simulink model "motorised_pid_bob_system"  (R2025b)
settings: Solver=FixedStepAuto  StartTime=0.0  StopTime=20  FixedStep=1e-4  RelTol=1e-3
values from neighbouring files (symbols this model uses):
  c = Simulink.Parameter    [motorised_BoB_system_with_PID.m]
  g = Simulink.Parameter    [motorised_BoB_system_with_PID.m]
  J_beam = Simulink.Parameter    [motorised_BoB_system_with_PID.m]
  J_motor = Simulink.Parameter    [dc_drives_system_parameter_declaraction.m]    (also in motorised_BoB_system_with_PID.m)
  k_e = Simulink.Parameter    [dc_drives_system_parameter_declaraction.m]    (also in motorised_BoB_system_with_PID.m)
  k_t = Simulink.Parameter    [dc_drives_system_parameter_declaraction.m]    (also in motorised_BoB_system_with_PID.m)
  KDpid = Simulink.Parameter    [motorised_BoB_system_with_PID.m]
  kFrs = Simulink.Parameter    [dc_drives_system_parameter_declaraction.m]
  KIpid = Simulink.Parameter    [motorised_BoB_system_with_PID.m]
  KPpid = Simulink.Parameter    [motorised_BoB_system_with_PID.m]
  L_a = Simulink.Parameter    [dc_drives_system_parameter_declaraction.m]    (also in motorised_BoB_system_with_PID.m)
  l_beam = Simulink.Parameter    [motorised_BoB_system_with_PID.m]
  m_ball = Simulink.Parameter    [motorised_BoB_system_with_PID.m]
  R_a = Simulink.Parameter    [dc_drives_system_parameter_declaraction.m]    (also in motorised_BoB_system_with_PID.m)
  r_ball = Simulink.Parameter    [motorised_BoB_system_with_PID.m]
  W_ci = Simulink.Parameter    [dc_drives_system_parameter_declaraction.m]
  W_cq = Simulink.Parameter    [dc_drives_system_parameter_declaraction.m]
  W_cw = Simulink.Parameter    [dc_drives_system_parameter_declaraction.m]
undefined symbols (not defined in the file or in its folder): L, R
settings Model: Creator=fycce  LastModifiedBy=fycce

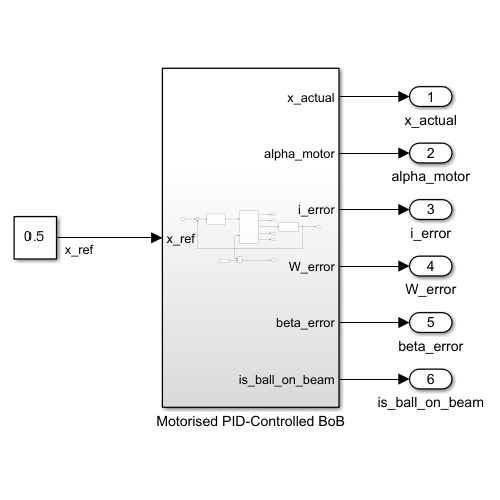
[thumbnail: Simulink's stored preview of the top-level diagram]
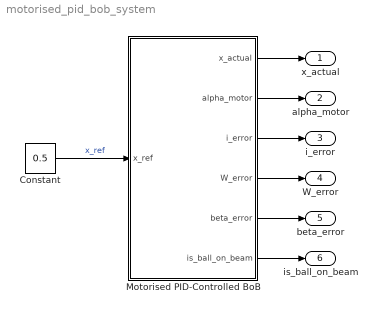
== system motorised_pid_bob_system ==
  Constant : Constant  Value=0.5
  Motorised PID-Controlled BoB : Subsystem
  x_actual : Outport
  alpha_motor : Outport  Port=2
  i_error : Outport  Port=3
  W_error : Outport  Port=4
  beta_error : Outport  Port=5
  is_ball_on_beam : Outport  Port=6
  wires:
  Constant/1 -> Motorised PID-Controlled BoB/1(x_ref)  "x_ref"
  Motorised PID-Controlled BoB/1(x_actual) -> x_actual/1
  Motorised PID-Controlled BoB/2(alpha_motor) -> alpha_motor/1
  Motorised PID-Controlled BoB/3(i_error) -> i_error/1
  Motorised PID-Controlled BoB/4(W_error) -> W_error/1
  Motorised PID-Controlled BoB/5(beta_error) -> beta_error/1
  Motorised PID-Controlled BoB/6(is_ball_on_beam) -> is_ball_on_beam/1

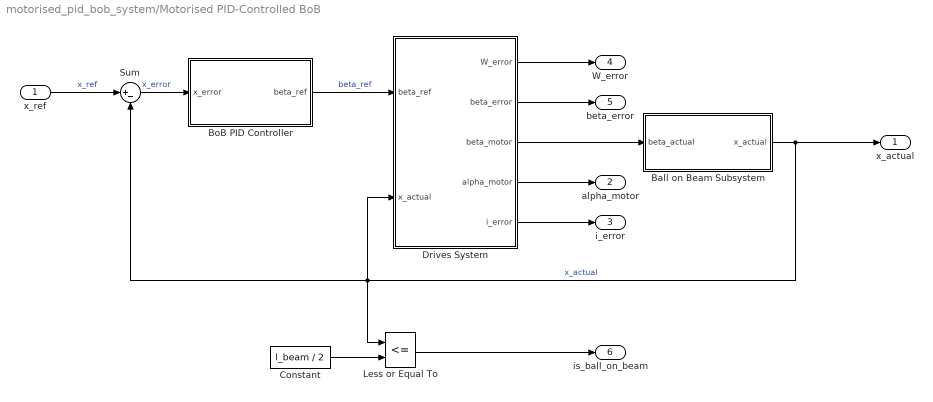
== system motorised_pid_bob_system/Motorised PID-Controlled BoB ==
  x_ref : Inport
  Ball on Beam Subsystem : Subsystem
  BoB PID Controller : Subsystem
  Constant : Constant  Value=l_beam / 2
  Drives System : Subsystem
  Less or Equal To : RelationalOperator  Operator=<=  OutDataTypeStr=boolean  RndMeth=Simplest  InputSameDT=off
  Sum : Sum  Inputs=|+-
  x_actual : Outport
  alpha_motor : Outport  Port=2
  i_error : Outport  Port=3
  W_error : Outport  Port=4
  beta_error : Outport  Port=5
  is_ball_on_beam : Outport  Port=6
  wires:
  Ball on Beam Subsystem/1(x_actual) -> x_actual/1, Less or Equal To/1, Sum/2, Drives System/2(x_actual)  "x_actual"
  Drives System/2(beta_error) -> beta_error/1
  Sum/1 -> BoB PID Controller/1(x_error)  "x_error"
  x_ref/1 -> Sum/1  "x_ref"
  Drives System/1(W_error) -> W_error/1
  Drives System/3(beta_motor) -> Ball on Beam Subsystem/1(beta_actual)
  Drives System/4(alpha_motor) -> alpha_motor/1
  BoB PID Controller/1(beta_ref) -> Drives System/1(beta_ref)  "beta_ref"
  Drives System/5(i_error) -> i_error/1
  Constant/1 -> Less or Equal To/2
  Less or Equal To/1 -> is_ball_on_beam/1

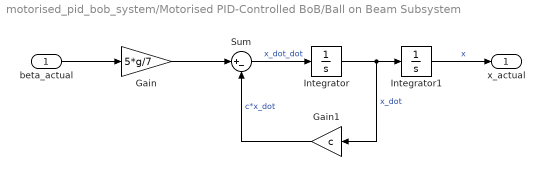
== system motorised_pid_bob_system/Motorised PID-Controlled BoB/Ball on Beam Subsystem ==
  beta_actual : Inport
  Gain : Gain  Gain=5*g/7
  Gain1 : Gain  Gain=c
  Integrator : Integrator
  Integrator1 : Integrator
  Sum : Sum  Inputs=|+-
  x_actual : Outport
  wires:
  Integrator1/1 -> x_actual/1  "x"
  beta_actual/1 -> Gain/1
  Integrator/1 -> Integrator1/1, Gain1/1  "x_dot"
  Gain/1 -> Sum/1
  Sum/1 -> Integrator/1  "x_dot_dot"
  Gain1/1 -> Sum/2  "c*x_dot"

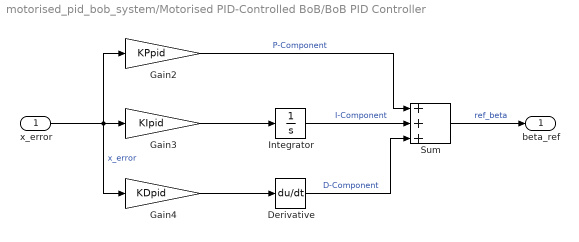
== system motorised_pid_bob_system/Motorised PID-Controlled BoB/BoB PID Controller ==
  x_error : Inport
  Derivative : Derivative
  Gain2 : Gain  Gain=KPpid
  Gain3 : Gain  Gain=KIpid
  Gain4 : Gain  Gain=KDpid
  Integrator : Integrator
  Sum : Sum  Inputs=+++
  beta_ref : Outport
  wires:
  Gain2/1 -> Sum/1  "P-Component"
  Integrator/1 -> Sum/2  "I-Component"
  Gain3/1 -> Integrator/1
  Sum/1 -> beta_ref/1  "ref_beta"
  Derivative/1 -> Sum/3  "D-Component"
  x_error/1 -> Gain4/1, Gain3/1, Gain2/1  "x_error"
  Gain4/1 -> Derivative/1

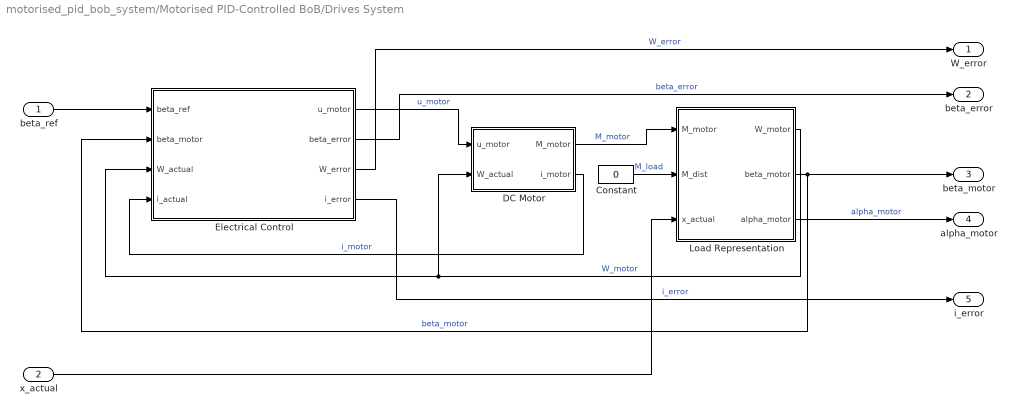
== system motorised_pid_bob_system/Motorised PID-Controlled BoB/Drives System ==
  beta_ref : Inport
  x_actual : Inport  Port=2
  Constant : Constant  Value=0
  DC Motor : Subsystem
  Electrical Control : Subsystem
  Load Representation : Subsystem
  W_error : Outport
  beta_error : Outport  Port=2
  beta_motor : Outport  Port=3
  alpha_motor : Outport  Port=4
  i_error : Outport  Port=5
  wires:
  DC Motor/2(i_motor) -> Electrical Control/4(i_actual)  "i_motor"
  Electrical Control/3(W_error) -> W_error/1  "W_error"
  Electrical Control/2(beta_error) -> beta_error/1  "beta_error"
  Load Representation/2(beta_motor) -> Electrical Control/2(beta_motor), beta_motor/1  "beta_motor"
  Electrical Control/1(u_motor) -> DC Motor/1(u_motor)  "u_motor"
  Load Representation/1(W_motor) -> Electrical Control/3(W_actual), DC Motor/2(W_actual)  "W_motor"
  DC Motor/1(M_motor) -> Load Representation/1(M_motor)  "M_motor"
  beta_ref/1 -> Electrical Control/1(beta_ref)
  Electrical Control/4(i_error) -> i_error/1  "i_error"
  Load Representation/3(alpha_motor) -> alpha_motor/1  "alpha_motor"
  Constant/1 -> Load Representation/2(M_dist)  "M_load"
  x_actual/1 -> Load Representation/3(x_actual)

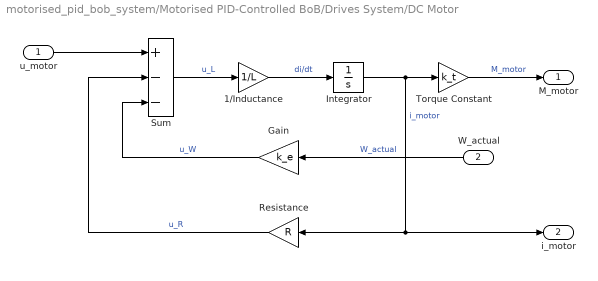
== system motorised_pid_bob_system/Motorised PID-Controlled BoB/Drives System/DC Motor ==
  u_motor : Inport
  W_actual : Inport  Port=2
  1/Inductance : Gain  Gain=1/L
  Gain : Gain  Gain=k_e
  Integrator : Integrator
  Resistance : Gain  Gain=R
  Sum : Sum  Inputs=+--
  Torque Constant : Gain  Gain=k_t
  M_motor : Outport
  i_motor : Outport  Port=2
  wires:
  u_motor/1 -> Sum/1
  Sum/1 -> 1/Inductance/1  "u_L"
  1/Inductance/1 -> Integrator/1  "di/dt"
  Integrator/1 -> i_motor/1, Resistance/1, Torque Constant/1  "i_motor"
  Torque Constant/1 -> M_motor/1  "M_motor"
  Resistance/1 -> Sum/2  "u_R"
  Gain/1 -> Sum/3  "u_W"
  W_actual/1 -> Gain/1  "W_actual"

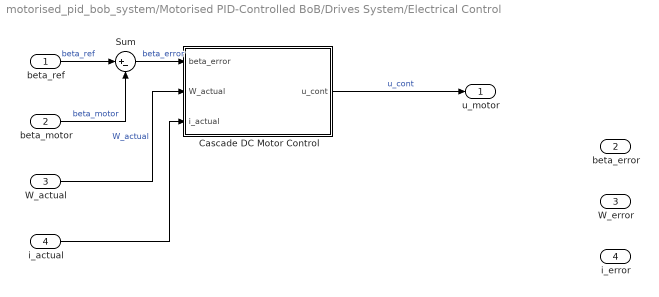
== system motorised_pid_bob_system/Motorised PID-Controlled BoB/Drives System/Electrical Control ==
  beta_ref : Inport
  beta_motor : Inport  Port=2
  W_actual : Inport  Port=3
  i_actual : Inport  Port=4
  Cascade DC Motor Control : Subsystem
  Sum : Sum  Inputs=|+-
  u_motor : Outport
  beta_error : Outport  Port=2
  W_error : Outport  Port=3
  i_error : Outport  Port=4
  wires:
  Cascade DC Motor Control/1(u_cont) -> u_motor/1  "u_cont"
  beta_ref/1 -> Sum/1  "beta_ref"
  beta_motor/1 -> Sum/2  "beta_motor"
  Sum/1 -> Cascade DC Motor Control/1(beta_error)  "beta_error"
  W_actual/1 -> Cascade DC Motor Control/2(W_actual)  "W_actual"
  i_actual/1 -> Cascade DC Motor Control/3(i_actual)

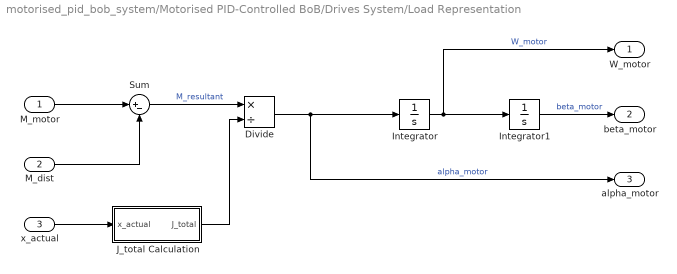
== system motorised_pid_bob_system/Motorised PID-Controlled BoB/Drives System/Load Representation ==
  M_motor : Inport
  M_dist : Inport  Port=2
  x_actual : Inport  Port=3
  Divide : Product  Inputs=*/
  Integrator : Integrator
  Integrator1 : Integrator
  J_total Calculation : Subsystem
  Sum : Sum  Inputs=|+-
  W_motor : Outport
  beta_motor : Outport  Port=2
  alpha_motor : Outport  Port=3
  wires:
  M_dist/1 -> Sum/2
  Sum/1 -> Divide/1  "M_resultant"
  Divide/1 -> Integrator/1, alpha_motor/1  "alpha_motor"
  Integrator/1 -> Integrator1/1, W_motor/1  "W_motor"
  Integrator1/1 -> beta_motor/1  "beta_motor"
  M_motor/1 -> Sum/1
  J_total Calculation/1(J_total) -> Divide/2
  x_actual/1 -> J_total Calculation/1(x_actual)

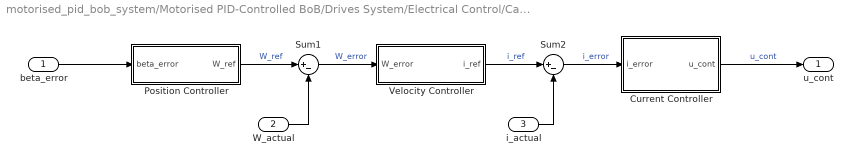
== system motorised_pid_bob_system/Motorised PID-Controlled BoB/Drives System/Electrical Control/Cascade DC Motor Control ==
  beta_error : Inport
  W_actual : Inport  Port=2
  i_actual : Inport  Port=3
  Current Controller : Subsystem
  Position Controller : Subsystem
  Sum1 : Sum  Inputs=|+-
  Sum2 : Sum  Inputs=|+-
  Velocity Controller : Subsystem
  u_cont : Outport
  wires:
  Position Controller/1(W_ref) -> Sum1/1  "W_ref"
  Sum1/1 -> Velocity Controller/1(W_error)  "W_error"
  Velocity Controller/1(i_ref) -> Sum2/1  "i_ref"
  Sum2/1 -> Current Controller/1(i_error)  "i_error"
  beta_error/1 -> Position Controller/1(beta_error)
  Current Controller/1(u_cont) -> u_cont/1  "u_cont"
  i_actual/1 -> Sum2/2
  W_actual/1 -> Sum1/2

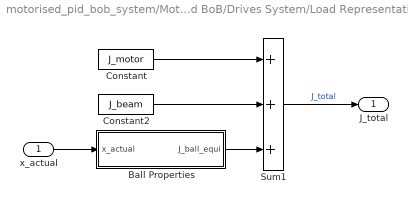
== system motorised_pid_bob_system/Motorised PID-Controlled BoB/Drives System/Load Representation/J_total Calculation ==
  x_actual : Inport
  Ball Properties : Subsystem
  Constant : Constant  Value=J_motor
  Constant2 : Constant  Value=J_beam
  Sum1 : Sum  Inputs=+++
  J_total : Outport
  wires:
  Constant2/1 -> Sum1/2
  Ball Properties/1(J_ball_equi) -> Sum1/3
  x_actual/1 -> Ball Properties/1(x_actual)
  Sum1/1 -> J_total/1  "J_total"
  Constant/1 -> Sum1/1

== system motorised_pid_bob_system/Motorised PID-Controlled BoB/Drives System/Electrical Control/Cascade DC Motor Control/Current Controller ==
  i_error : Inport
  Gain : Gain  Gain=L_a*W_ci
  Gain2 : Gain  Gain=R_a*W_ci
  Integrator : Integrator
  Sum1 : Sum  Inputs=|++
  u_cont : Outport
  wires:
  Gain2/1 -> Integrator/1
  Gain/1 -> Sum1/1
  Integrator/1 -> Sum1/2
  i_error/1 -> Gain2/1, Gain/1
  Sum1/1 -> u_cont/1

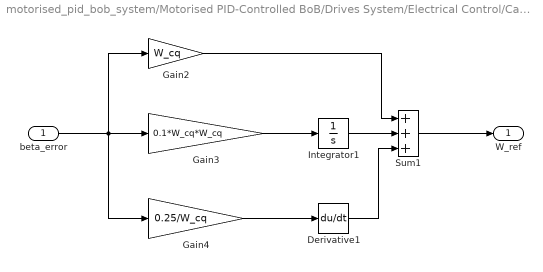
== system motorised_pid_bob_system/Motorised PID-Controlled BoB/Drives System/Electrical Control/Cascade DC Motor Control/Position Controller ==
  beta_error : Inport
  Derivative1 : Derivative
  Gain2 : Gain  Gain=W_cq
  Gain3 : Gain  Gain=0.1*W_cq*W_cq
  Gain4 : Gain  Gain=0.25/W_cq
  Integrator1 : Integrator
  Sum1 : Sum  Inputs=+++
  W_ref : Outport
  wires:
  Sum1/1 -> W_ref/1
  beta_error/1 -> Gain3/1, Gain4/1, Gain2/1
  Gain2/1 -> Sum1/1
  Derivative1/1 -> Sum1/3
  Integrator1/1 -> Sum1/2
  Gain3/1 -> Integrator1/1
  Gain4/1 -> Derivative1/1

== system motorised_pid_bob_system/Motorised PID-Controlled BoB/Drives System/Electrical Control/Cascade DC Motor Control/Velocity Controller ==
  W_error : Inport
  I-Gain : Gain  Gain=kFrs*W_cw/k_t
  Integrator : Integrator
  P-Gain : Gain  Gain=(J_motor + J_beam+2/5*m_ball*r_ball*r_ball)*W_cw/k_t
  Sum : Sum  Inputs=|++
  i_ref : Outport
  wires:
  W_error/1 -> I-Gain/1, P-Gain/1  "W_error"
  I-Gain/1 -> Integrator/1
  Sum/1 -> i_ref/1  "i_ref"
  P-Gain/1 -> Sum/1  "i_P"
  Integrator/1 -> Sum/2  "i_I"

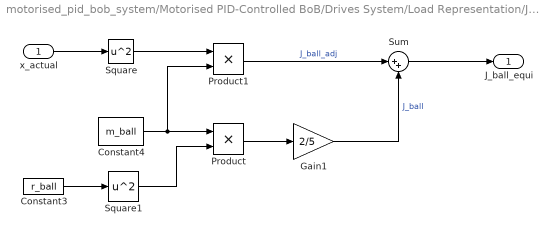
== system motorised_pid_bob_system/Motorised PID-Controlled BoB/Drives System/Load Representation/J_total Calculation/Ball Properties ==
  x_actual : Inport
  Constant3 : Constant  Value=r_ball
  Constant4 : Constant  Value=m_ball
  Gain1 : Gain  Gain=2/5
  Product : Product
  Product1 : Product
  Square : Math  Operator=square
  Square1 : Math  Operator=square
  Sum : Sum  Inputs=|++
  J_ball_equi : Outport
  wires:
  Square1/1 -> Product/2
  Constant4/1 -> Product1/2, Product/1
  Constant3/1 -> Square1/1
  Square/1 -> Product1/1
  x_actual/1 -> Square/1
  Product/1 -> Gain1/1
  Product1/1 -> Sum/1  "J_ball_adj"
  Gain1/1 -> Sum/2  "J_ball"
  Sum/1 -> J_ball_equi/1
